simulink model "controller"  (R2023b)
settings: Solver=VariableStepAuto  StartTime=0.0  StopTime=1  MaxStep=1e-5  RelTol=1e-3
undefined symbols (not defined in the file): A, accDir, B, C, K_i, K_r, ke, L, p, p0, targetPos, v0
settings Model: Creator=miqui  LastModifiedBy=miqui

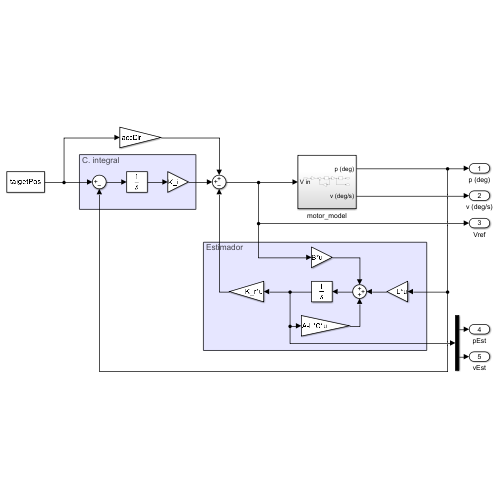
[thumbnail: Simulink's stored preview of the top-level diagram]
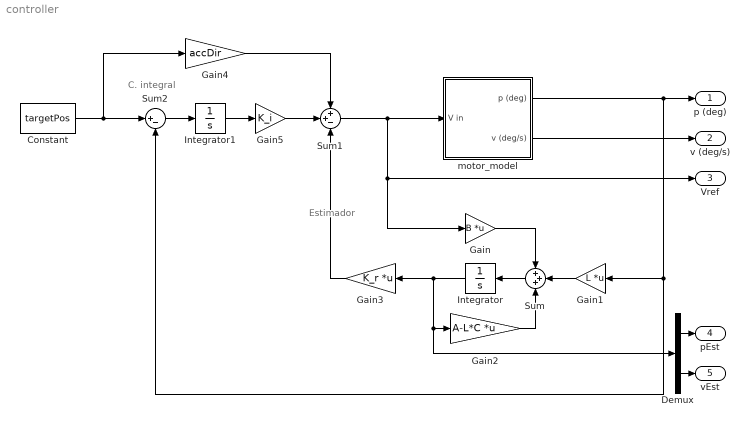
== system controller ==
  note: Estimador
  note: C. integral
  Constant : Constant  Value=targetPos
  Demux : Demux  Outputs=2
  Gain : Gain  Gain=B  Multiplication=Matrix(K*u)
  Gain1 : Gain  Gain=L  Multiplication=Matrix(K*u)
  Gain2 : Gain  Gain=A-L*C  Multiplication=Matrix(K*u)
  Gain3 : Gain  Gain=K_r  Multiplication=Matrix(K*u)
  Gain4 : Gain  Gain=accDir
  Gain5 : Gain  Gain=K_i
  Integrator : Integrator
  Integrator1 : Integrator
  Sum : Sum  Inputs=+++
  Sum1 : Sum  Inputs=++-
  Sum2 : Sum  Inputs=|+-
  motor_model : Subsystem
  p (deg) : Outport
  v (deg/s) : Outport  Port=2
  Vref : Outport  Port=3
  pEst : Outport  Port=4
  vEst : Outport  Port=5
  wires:
  Sum/1 -> Integrator/1
  Gain/1 -> Sum/1
  Gain1/1 -> Sum/2
  Gain2/1 -> Sum/3
  Integrator/1 -> Demux/1, Gain2/1, Gain3/1
  Gain3/1 -> Sum1/3
  Sum1/1 -> motor_model/1(V in), Vref/1, Gain/1
  Gain4/1 -> Sum1/1
  Sum2/1 -> Integrator1/1
  Integrator1/1 -> Gain5/1
  Gain5/1 -> Sum1/2
  Constant/1 -> Sum2/1, Gain4/1
  motor_model/1(p (deg)) -> p (deg)/1, Gain1/1, Sum2/2
  motor_model/2(v (deg/s)) -> v (deg/s)/1
  Demux/1 -> pEst/1
  Demux/2 -> vEst/1

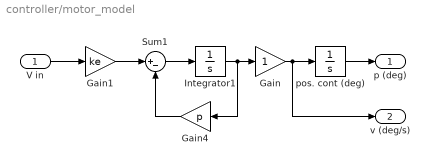
== system controller/motor_model ==
  V in : Inport
  Gain : Gain
  Gain1 : Gain  Gain=ke
  Gain4 : Gain  Gain=p
  Integrator1 : Integrator  InitialCondition=v0
  Sum1 : Sum  Inputs=|+-
  pos. cont (deg) : Integrator  InitialCondition=p0
  p (deg) : Outport
  v (deg/s) : Outport  Port=2
  wires:
  Sum1/1 -> Integrator1/1
  Gain4/1 -> Sum1/2
  Integrator1/1 -> Gain/1, Gain4/1
  Gain1/1 -> Sum1/1
  Gain/1 -> pos. cont (deg)/1, v (deg/s)/1
  pos. cont (deg)/1 -> p (deg)/1
  V in/1 -> Gain1/1
